simulink model "impulseorder1type0"  (R2018b)
settings: Solver=VariableStepAuto  StartTime=0.0  StopTime=10.0  RelTol=1e-3
libraries: simulink_extras x3
settings Model: Creator=Ratish Kumar S  LastModifiedBy=Ratish Kumar S

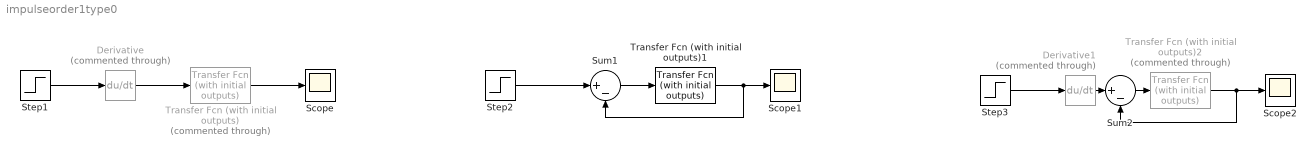
== system impulseorder1type0 ==
  Derivative : Derivative  Commented=through
  Derivative1 : Derivative  Commented=through
  Scope : Scope
  Scope1 : Scope
  Scope2 : Scope
  Step1 : Step  Time=0  After=10  SampleTime=0
  Step2 : Step  Time=0  After=10  SampleTime=0
  Step3 : Step  Time=0  After=10  SampleTime=0
  Sum1 : Sum  Inputs=|+-
  Sum2 : Sum  Inputs=|+-
  Transfer Fcn (with initial outputs) : simulink_extras/Additional Linear/Transfer Fcn (with initial outputs)  Commented=through  N=[4]  D="[1  2]"  Y0=.5  U0=0
  Transfer Fcn (with initial outputs)1 : simulink_extras/Additional Linear/Transfer Fcn (with initial outputs)  N=[4]  D="[1  2]"  Y0=.5  U0=0
  Transfer Fcn (with initial outputs)2 : simulink_extras/Additional Linear/Transfer Fcn (with initial outputs)  Commented=through  N=[4]  D="[1  2]"  Y0=.5  U0=0
  wires:
  Step1/1 -> Derivative/1
  Derivative/1 -> Transfer Fcn (with initial outputs)/1
  Transfer Fcn (with initial outputs)/1 -> Scope/1
  Step2/1 -> Sum1/1
  Transfer Fcn (with initial outputs)1/1 -> Scope1/1, Sum1/2
  Sum1/1 -> Transfer Fcn (with initial outputs)1/1
  Transfer Fcn (with initial outputs)2/1 -> Sum2/2, Scope2/1
  Step3/1 -> Derivative1/1
  Derivative1/1 -> Sum2/1
  Sum2/1 -> Transfer Fcn (with initial outputs)2/1
